simulink model "Schimmel_Evan_lab_1_model"  (R2020b)
settings: Solver=VariableStepAuto  StartTime=0.0  StopTime=tf  MaxStep=maxstep  RelTol=tol  AbsTol=tol
values from neighbouring files (symbols this model uses):
  c = 1    [Schimmel_Evan_lab_1_script.m]
  F = 10    [BlockDragM.m]    (also in Schimmel_Evan_lab_1_script.m = 6)
  k = 20    [Schimmel_Evan_lab_1_script.m]
  m = 1    [BlockDragM.m]    (also in Schimmel_Evan_lab_1_script.m = 2)
  v0 = 1    [BlockDragM.m]    (also in Schimmel_Evan_lab_1_script.m = -1)
  x0 = 0.2    [Schimmel_Evan_lab_1_script.m]
settings Model: Creator=schimmer  LastModifiedBy=schimmer
settings DataIOCC: SaveOutput=off  SignalLogging=off  DSMLogging=off  SaveTime=off  ReturnWorkspaceOutputs=off

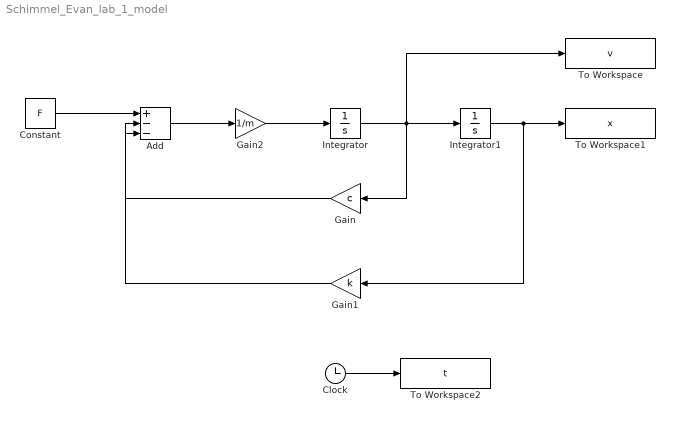
== system Schimmel_Evan_lab_1_model ==
  Add : Sum  Inputs=+--
  Clock : Clock
  Constant : Constant  Value=F
  Gain : Gain  Gain=c
  Gain1 : Gain  Gain=k
  Gain2 : Gain  Gain=1/m
  Integrator : Integrator  InitialCondition=v0
  Integrator1 : Integrator  InitialCondition=x0
  To Workspace : ToWorkspace  VariableName=v  SampleTime=-1
  To Workspace1 : ToWorkspace  VariableName=x  SampleTime=-1
  To Workspace2 : ToWorkspace  VariableName=t  SampleTime=-1
  wires:
  Integrator/1 -> To Workspace/1, Integrator1/1, Gain/1
  Integrator1/1 -> Gain1/1, To Workspace1/1
  Add/1 -> Gain2/1
  Gain2/1 -> Integrator/1
  Gain1/1 -> Add/2
  Gain/1 -> Add/3
  Constant/1 -> Add/1
  Clock/1 -> To Workspace2/1
